simulink model "Irradiance__"  (R2024b)
settings: Solver=ode23  StartTime=0.0  StopTime=1200  RelTol=1e-3
values from neighbouring files (symbols this model uses):
  CellNum = 54    [Inititialisation.m]
  E_g = 1.1    [Inititialisation.m]
  G_ref = 1000    [Inititialisation.m]
  I_sc = 8.21    [Inititialisation.m]
  k_Boltz = 1.380649e-23    [Inititialisation.m]
  K_Isc = 0.0032    [Inititialisation.m]
  K_Vsc = -0.1230    (= -0.123)    [Inititialisation.m]
  LookupR = readmatrix("Data_Out.xlsx", Sheet="Lookup")    [Inititialisation.m]
  n = 0.64611    [Inititialisation.m]
  Num_Paral = 1    [Inititialisation.m]
  NumSeries = 1    [Inititialisation.m]
  q = 1.60217663e-19    [Inititialisation.m]
  R_p = 65.4647    [Inititialisation.m]
  R_s = 0.47804    [Inititialisation.m]
  T_ref = 25+273.15    (= 298.15)    [Inititialisation.m]
  V_oc = 32.9    [Inititialisation.m]
undefined symbols (not defined in the file or in its folder): X, Y, Z
libraries: simulink_extras x10, WormAndGearConstraintLibrary x6, sm_lib x4, nesl_utility x3, fl_lib x2, SignalEditorBlockLib x1
settings Model: Creator=Harrison  LastModifiedBy=Harrison
settings SolverCC: ZeroCrossAlgorithm=Adaptive
settings DebuggingCC: IgnoredZcDiagnostic=none
settings ExplorerConfigSet: InternalSimMechanicsExplorerSettings="<ExplorerConfiguration><canonicalview>default</canonicalview><AnimationSetting><BasePlaybackSpeed>1.0</BasePlaybackSpeed><PlaybackSpeedFactor>0.00390625</PlaybackSpeedFactor></AnimationSetting><TilePanel><TileInfo><Tiles Columns=\"1\" Count=\"1\" Rows=\"1\"><Column Weight=\"1\"/><Row Weight=\"1\"/><Tile Height=\"1\" Width=\"1\" X=\"0\" Y=\"0\"/></Tiles></TileInfo><SceneInfo><SceneViewer><BGColor><R>0.60000002384185791</R><G>0.60000002384185791</G><B>0.60000002384185791</B></BGColor><Camera><DoPerspective>off</DoPerspective><Position><X>0.904674596207072468</X><Y>-1.01398600552732976</Y><Z>1.30819149571960591</Z></Position><Center><X>0.0315254730978809794</X><Y>0.0558159470207882369</Y><Z>0.923626353226344343</Z></Center><Up><X>-0.146611699468769036</X><Y>0.226481916389170257</Y><Z>0.962917935821930748</Z></Up><ViewLimDist>1</ViewLimDist><YLim>0.98754073208570492</YLim><XLim>0.758290204994380601</XLim></Camera></SceneViewer></SceneInfo></TilePanel><MechEditorPanel><Cameras/><GfxPanelCameraMap/><VideoCreator><PlaybackSpeedRatio>0.00115740</PlaybackSpeedRatio><FrameRate>60</FrameRate><VideoFormat>MPEG-4</VideoFormat><FrameSize>auto</FrameSize></VideoCreator></MechEditorPanel></ExplorerConfiguration>"

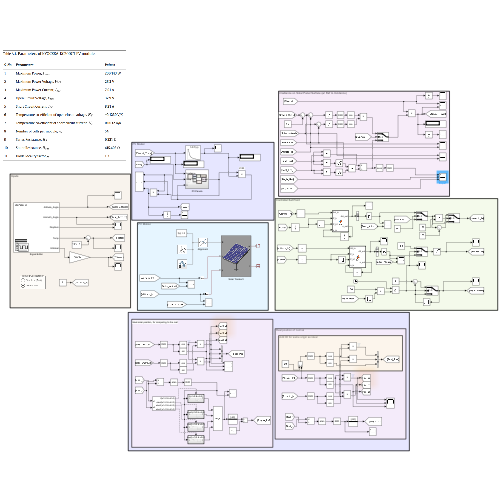
[thumbnail: Simulink's stored preview of the top-level diagram]
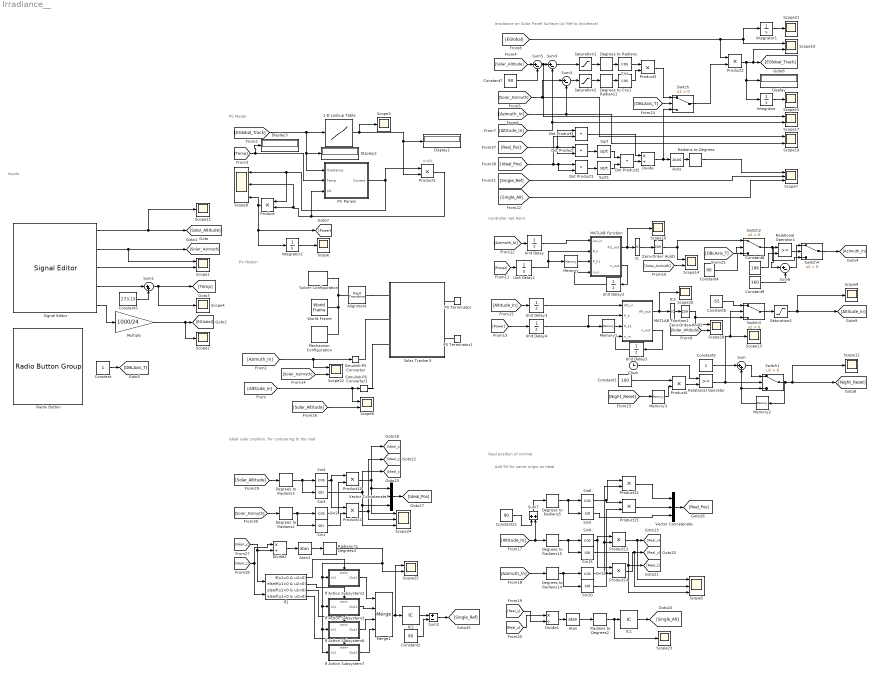
== system Irradiance__ ==
  note: Irradiance on Solar Panel Surface (w/ Ref to Incidence)
  note: Controller Set Point
  note: V=IR
  note: Inputs
  note: PV Motion
  note: PV Model
  note: Ideal solar position, for comparing to the real
  note: Add 90 for same origin as ideal
  note: Real position of normal
  1-D Lookup Table : Lookup_n-D  NumberOfTableDimensions=1  BreakpointsForDimension1=[LookupR(:,1)]  Table=[LookupR(:,2)]  InternalRulePriority=Speed  RndMeth=Simplest
  Acos : Trigonometry  Operator=acos
  Alignment : sm_lib/Frames and Transforms/Rigid Transform  RotationMethod=AlignedAxes  FollAlignAxisA=+Z  BaseAlignAxisA=+Z  FollAlignAxisB=+Y  BaseAlignAxisB=-X  RotationStandardAxis=+Z  RotationAngle=0.0  RotationAngleUnits=deg  RotationArbitraryAxis=[0 0 1]  RotationSequenceAxes=FollowerAxes  RotationSequence=XYX  RotationSequenceAngles=[0 0 0]  RotationSequenceAnglesUnits=deg  RotationMatrix=[1 0 0; 0 1 0; 0 0 1]  Quaternion=[1 0 0 0]  TranslationMethod=None  TranslationCartesianOffset=[0 0 0]  TranslationCartesianOffsetUnits=m  TranslationStandardAxis=+Z  TranslationStandardOffset=0  TranslationStandardOffsetUnits=m  TranslationROffset=0  TranslationROffsetUnits=m  TranslationThetaOffset=0  TranslationThetaOffsetUnits=deg  TranslationZOffset=0  TranslationZOffsetUnits=m
  Atan : Trigonometry  Operator=atan
  Atan1 : Trigonometry  Operator=atan
  Clock : Clock
  Constant : Constant
  Constant1 : Constant  Value=100
  Constant{2,4,7,21} (4 alike) : Constant  Value=90
  Constant3 : Constant  Value=273.15
  Constant5 : Constant
  Constant6 : Constant  Value=-55
  Constant8 : Constant  Value=186
  Constant9 : Constant  Value=360
  Cos : Trigonometry  Operator=cos
  Cos1 : Trigonometry  Operator=cos
  Degrees to Radians{,1..3,5,14..15} (7 alike) : simulink_extras/Transformations/Degrees to Radians
  Display{,1..3} (4 alike) : Display
  Divide : Product  Inputs=*/
  Divide1 : Product  Inputs=*/
  Divide2 : Product  Inputs=*/
  Dot Product{,1..3} (4 alike) : DotProduct  OutDataTypeStr=Inherit: Inherit via internal rule
  IC : InitialCondition  Value=0
  IC1 : InitialCondition  Value=-60
  IC2 : InitialCondition  Value=-60
  IC3 : InitialCondition  Value=-60
  If Action Subsystem2 : Subsystem  TreatAsAtomicUnit=on
  If Action Subsystem3 : Subsystem  TreatAsAtomicUnit=on
  If Action Subsystem6 : Subsystem  TreatAsAtomicUnit=on
  If Action Subsystem7 : Subsystem  TreatAsAtomicUnit=on
  If1 : If  NumInputs=2  IfExpression=u1>0 & u2>0  ElseIfExpressions=u1>0 & u2<0, u1<0 & u2<0, u1<0 & u2>0  ShowElse=off
  Integrator : Integrator
  Integrator1 : Integrator
  Integrator2 : Integrator
  MATLAB Function : MATLAB Function  TreatAsAtomicUnit=on
  MATLAB Function1 : MATLAB Function  TreatAsAtomicUnit=on
  Mechanism Configuration : sm_lib/Utilities/Mechanism Configuration  UniformGravity=Constant  GravityVector=[0 0 -9.80665]  GravityVectorUnits=m/s^2  LinearizationDelta=0.001  JointModeTransitionNonlinearIterations=2
  Memory : Memory
  Memory1 : Memory
  Memory2 : Memory  InitialCondition=1
  Memory3 : Memory  InitialCondition=1
  Merge1 : Merge  Inputs=4
  Multiply : Gain  Gain=1000/24
  PS Terminator : fl_lib/Physical Signals/Sinks/PS Terminator
  PS Terminator1 : fl_lib/Physical Signals/Sinks/PS Terminator
  PV Panels : Subsystem
  Product{,1..4,10..15} (11 alike) : Product
  Radians to Degrees : simulink_extras/Transformations/Radians to Degrees
  Radians to Degrees2 : simulink_extras/Transformations/Radians to Degrees
  Radians to Degrees3 : simulink_extras/Transformations/Radians to Degrees
  Radio Button : RadioButtonGroup  LabelPosition=Hide  SelectedLabel=Double Axis  ButtonGroupName=Tracking Configuration
      settings: Values={{'One Axis (E-W)', 'Double Axis'}, [0 1]}
  Relational Operator : RelationalOperator  OutDataTypeStr=boolean  RndMeth=Simplest  InputSameDT=off
  Relational Operator1 : RelationalOperator  OutDataTypeStr=boolean  RndMeth=Simplest  InputSameDT=off
  Saturation1 : Saturate  UpperLimit=90  LowerLimit=-90
  Saturation2 : Saturate  UpperLimit=90  LowerLimit=-90
  Saturation4 : Saturate  UpperLimit=60  LowerLimit=-60
  Scope{,2..4,9,11..13,15..16,20..21,23} (13 alike) : Scope
  Scope{1,6,10,14,17..19,22,25} (9 alike) : Scope  NumInputPorts=2
  Scope{5,7..8,24} (4 alike) : Scope  NumInputPorts=3
  Signal Editor : SignalEditorBlockLib/Signal Editor  FileName=C:\Users\Harrison\OneDrive\Documents\from 2021\Uni\University\Year 3\Final Year Project\Models\SimOutputs\All_Scenario.mat  ActiveScenario=Scenario_3  ActiveSignal=Altitude_Angle  IsBus=off  OutputBusObjectStr=Bus: BusObject  SampleTime=0  Interpolate=off  ZeroCross=off  OutputAfterFinalValue=Setting to zero  Unit=inherit  PreserveSignalName=on  ApplySigPropsToAllScenarios=on  ApplySigPropsToAllSignals=off
  Simulink-PS Converter : nesl_utility/Simulink-PS Converter  PhysicalDomain=network_engine_domain  SubClassName=ps_input  LeftPortType=input  RightPortType=output  PseudoPeriodic=off  Frequencies=[]  NoiseDistribution=none  NoiseParameters=[]  Unit=deg  AffineConversion=off  FilteringAndDerivatives=filter  SimscapeFilterOrder=2  InputFilterTimeConstant=0.001  UdotUserProvided=0
  Simulink-PS Converter1 : nesl_utility/Simulink-PS Converter  PhysicalDomain=network_engine_domain  SubClassName=ps_input  LeftPortType=input  RightPortType=output  PseudoPeriodic=off  Frequencies=[]  NoiseDistribution=none  NoiseParameters=[]  Unit=deg  AffineConversion=off  FilteringAndDerivatives=filter  SimscapeFilterOrder=2  InputFilterTimeConstant=0.001  UdotUserProvided=0
  Sin{1,3,5,10,15} (5 alike) : Trigonometry
  Sin{2,4,6,9,11} (5 alike) : Trigonometry  Operator=cos
  Solar Tracker3 : Subsystem
      mask Display:
      | image(fullfile('WormAndGearConstraintSupport','Images','SolarTracker.png'));
      | port_label('lconn',1,'B');
      | port_label('lconn',2,'y');
      | port_label('lconn',3,'p');
      | port_label('rconn',1,'w');
      | port_label('rconn',2,'t');
  Solver Configuration : nesl_utility/Solver Configuration  PhysicalDomain=network_engine_domain  SubClassName=solver  LeftPortType=input  RightPortType=generic  Tones=[]  Harmonics=[]  SimulateNoise=off  Profile=off  UseLocalSampling=off  EnableSwitchedLinearOptims=on  FrequencyDomain=off  UseCCode=off  RelTol=0.001  AbsTol=1e-06  MinStep=1e-09  ToWorkspace=off  RevertToSquareIcSolve=off  NumHomotopyIterations=100  PhasorMode=off  PhasorModeNumHarmonics=1  ConsistencySolver=NEWTON_FTOL  IndexReductionMethod=DerivativeReplacement  DoDC=off  ResidualTolerance=1e-09  ConsistencyTolSource=GLOBAL  ConsistencyAbsTol=0.001  ConsistencyRelTol=0.001  ConsistencyTolFactor=0.001  UseLocalSolver=off  LocalSolverChoice=NE_BACKWARD_EULER_ADVANCER  ResolveIndetEquations=on  FunctionEvalNumThread=1  LocalSolverSampleTime=0.001  DoFixedCost=off  MaxNonlinIter=3  MaxModeIter=2  ComputeImpulses=off  ImpulseIterations=2  LinearAlgebra=Sparse  LinearAlgebraNumThread=0  EquationFormulation=NE_TIME_EF  DelaysMemoryBudget=1024  AutomaticFiltering=on  FilteringTimeConstant=0.001  PartitionStorageMethod=AS_NEEDED  PartitionMemoryBudget=1024  PartitionMethod=FAST  MultibodyUseLocalSolver=off  MultibodyLocalSolverChoice=ODE1  MultibodyLocalSolverSampleTime=0.001
  Sqrt : Sqrt
  Sqrt1 : Sqrt
  Sum : Sum  Inputs=|++
  Sum1 : Sum  Inputs=|++
  Sum2 : Sum  Inputs=+-
  Sum{3..6} (4 alike) : Sum  Inputs=|+-
  Sum7 : Sum
  Switch{,1..4} (5 alike) : Switch  Criteria=u2 > Threshold  SaturateOnIntegerOverflow=off  InputSameDT=off
  Unit Delay : UnitDelay  SampleTime=0.015  HasFrameUpgradeWarning=on
  Unit Delay1 : UnitDelay  SampleTime=0.015  HasFrameUpgradeWarning=on
  Unit Delay2 : UnitDelay  SampleTime=0.015  HasFrameUpgradeWarning=on
  Unit Delay3 : UnitDelay  SampleTime=0.01  HasFrameUpgradeWarning=on
  Unit Delay4 : UnitDelay  SampleTime=0.01  HasFrameUpgradeWarning=on
  Unit Delay5 : UnitDelay  SampleTime=0.01  HasFrameUpgradeWarning=on
  Vector Concatenate : Concatenate  NumInputs=3
  Vector Concatenate1 : Concatenate  NumInputs=3
  World Frame : sm_lib/Frames and Transforms/World Frame
  Zero-Order Hold1 : ZeroOrderHold  SampleTime=0.015
  Zero-Order Hold2 : ZeroOrderHold  SampleTime=0.01
  wires:
  Product1/1 -> PV Panels/3(In1), Scope8/2, Product/2
  PV Panels/1(Current) -> Product1/1, Product/1, Scope8/1
  Constant3/1 -> Sum1/2
  [Azimuth_In] -> Scope22/1, Simulink-PS Converter/1
  Multiply/1 -> [EGlobal], Scope2/1
  Sum1/1 -> [Temp], Scope4/1
  [EGlobal_Track] -> 1-D Lookup Table/1, Display2/1, PV Panels/1(Irradiance)
  [Temp] -> Display3/1, PV Panels/2(Temp)
  Signal Editor/2 -> [Solar_Azimuth], Scope1/1
  Signal Editor/3 -> Scope1/2
  Signal Editor/5 -> Multiply/1
  Signal Editor/4 -> Sum1/1
  1-D Lookup Table/1 -> Scope3/1, Product1/2, Display1/1
  Cos/1 -> Product3/1
  Cos1/1 -> Product3/2
  [EGlobal] -> Integrator1/1, Scope10/1, Product2/1
  Degrees to Radians/1 -> Cos/1
  Degrees to Radians1/1 -> Cos1/1
  Memory/1 -> MATLAB Function/3(P_k1)
  MATLAB Function/1(Azi_out) -> Scope16/1, IC/1
  Product/1 -> Integrator2/1, [Power], Scope8/3
  Product2/1 -> Scope10/2, [EGlobal_Track], Integrator/1, Display/1
  [Solar_Azimuth] -> Sum4/1, Scope19/1
  [Azimuth_In] -> Scope19/2, Sum4/2
  [Altitude_In] -> Sum3/2, Scope17/2
  Signal Editor/1 -> Scope11/1, [Solar_Altitude]
  Sum4/1 -> Saturation2/1
  Sum3/1 -> Saturation1/1
  Saturation2/1 -> Degrees to Radians1/1
  Saturation1/1 -> Degrees to Radians/1
  Unit Delay2/1 -> MATLAB Function/4(n_in)
  Unit Delay5/1 -> MATLAB Function1/4(n_in)
  MATLAB Function1/1(Alt_out) -> IC3/1, Scope20/1
  Memory1/1 -> MATLAB Function1/3(P_k1)
  [Altitude_In] -> Scope6/1, Simulink-PS Converter1/1
  [Azimuth_In] -> Unit Delay/1
  Unit Delay/1 -> MATLAB Function/1(Azi_in)
  Unit Delay1/1 -> MATLAB Function/2(P_k), Memory/1
  MATLAB Function/2(n_out) -> Unit Delay2/1
  [Power] -> Unit Delay1/1
  IC/1 -> Zero-Order Hold1/1
  Zero-Order Hold1/1 -> Scope14/1, Switch2/1
  [Solar_Azimuth] -> Scope14/2
  [Power] -> Unit Delay4/1
  Unit Delay4/1 -> MATLAB Function1/2(P_k), Memory1/1
  MATLAB Function1/2(n_out) -> Unit Delay5/1
  IC3/1 -> Zero-Order Hold2/1
  [Solar_Altitude] -> Scope18/2
  [Solar_Azimuth] -> Scope22/2
  [Solar_Altitude] -> Scope6/2
  [Real_y] -> Divide1/2
  [Ideal_y] -> Divide2/2, If1/1
  [Azimuth_In] -> Degrees to Radians14/1
  If Action Subsystem3/1(Out1) -> Merge1/2
  Degrees to Radians2/1 -> Sin2/1, Sin1/1
  Atan1/1 -> Radians to Degrees3/1
  Constant21/1 -> Sum7/1
  If Action Subsystem2/1(Out1) -> Merge1/1
  Merge1/1 -> IC2/1, Scope25/1
  Divide2/1 -> Atan1/1
  Radians to Degrees2/1 -> IC1/1, Scope23/1
  Product15/1 -> Vector Concatenate/2
  Divide1/1 -> Atan/1
  Vector Concatenate1/1 -> [Ideal_Pos]
  If Action Subsystem7/1(Out1) -> Merge1/4
  IC2/1 -> Sum2/1
  [Solar_Altitude] -> Degrees to Radians3/1
  Product13/1 -> Scope5/1, [Real_x]
  [Real_z] -> Divide1/1
  Sum7/1 -> Degrees to Radians5/1
  If1/3 -> If Action Subsystem6/Action
  Sin9/1 -> Product13/1, Product14/1
  [Solar_Azimuth] -> Degrees to Radians2/1
  Degrees to Radians15/1 -> Sin15/1, Sin9/1
  Sin3/1 -> Scope24/3, Vector Concatenate1/3, [Ideal_z]
  If Action Subsystem6/1(Out1) -> Merge1/3
  Radians to Degrees3/1 -> If Action Subsystem2/1(In1), If Action Subsystem3/1(In1), If Action Subsystem6/1(In1), If Action Subsystem7/1(In1), Scope25/2
  Sin11/1 -> Product13/2, Product12/2
  [Ideal_z] -> Divide2/1, If1/2
  Product12/1 -> Vector Concatenate/1
  If1/2 -> If Action Subsystem3/Action
  Product11/1 -> [Ideal_y], Vector Concatenate1/2, Scope24/2
  Atan/1 -> Radians to Degrees2/1
  Degrees to Radians5/1 -> Sin6/1, Sin5/1
  Sin1/1 -> Product11/2
  Product14/1 -> Scope5/2, [Real_y]
  Sum2/1 -> [Single_Ref]
  Sin15/1 -> Scope5/3, [Real_z]
  If1/4 -> If Action Subsystem7/Action
  Sin4/1 -> Product11/1, Product10/1
  Sin10/1 -> Product15/2, Product14/2
  Degrees to Radians3/1 -> Sin4/1, Sin3/1
  IC1/1 -> [Single_Alt]
  If1/1 -> If Action Subsystem2/Action
  Constant2/1 -> Sum2/2
  Sin5/1 -> Vector Concatenate/3
  Degrees to Radians14/1 -> Sin10/1, Sin11/1
  Sin2/1 -> Product10/2
  [Altitude_In] -> Sum7/2, Degrees to Radians15/1
  Product10/1 -> Vector Concatenate1/1, Scope24/1, [Ideal_x]
  Sin6/1 -> Product15/1, Product12/1
  Vector Concatenate/1 -> [Real_Pos]
  Sqrt1/1 -> Dot Product2/2
  Dot Product3/1 -> Divide/1
  Dot Product/1 -> Sqrt/1
  [Ideal_Pos] -> Dot Product3/2, Dot Product1/1, Dot Product1/2
  Dot Product1/1 -> Sqrt1/1
  Dot Product2/1 -> Divide/2
  Sqrt/1 -> Dot Product2/1
  [Real_Pos] -> Dot Product3/1, Dot Product/2, Dot Product/1
  Product3/1 -> Switch/1
  Switch/1 -> Product2/2
  Divide/1 -> Switch/3, Acos/1
  [DBLAxis_T] -> Switch/2
  Acos/1 -> Radians to Degrees/1
  Radians to Degrees/1 -> Scope7/1
  [Single_Ref] -> Scope7/2
  [Single_Alt] -> Scope7/3
  Constant/1 -> [DBLAxis_T]
  [Altitude_In] -> Unit Delay3/1
  Unit Delay3/1 -> MATLAB Function1/1(Alt_in)
  Zero-Order Hold2/1 -> Scope18/1, Switch3/3
  Constant4/1 -> Switch2/3
  [DBLAxis_T] -> Switch2/2
  Switch2/1 -> Switch4/3, Sum6/1, Relational Operator1/1
  Constant1/1 -> Product4/1
  Product4/1 -> Relational Operator/2
  Clock/1 -> Relational Operator/1
  Constant5/1 -> Sum/1
  Switch1/1 -> Memory2/1, Scope12/1, [Night_Reset]
  Memory2/1 -> Switch1/3, Sum/2
  Sum/1 -> Switch1/1
  [Night_Reset] -> Memory3/1
  Relational Operator/1 -> Switch1/2, Scope13/1, Switch3/2
  Memory3/1 -> Product4/2
  Switch3/1 -> Saturation4/1
  Constant6/1 -> Switch3/1
  Saturation4/1 -> Scope9/1, [Altitude_In]
  Sum5/1 -> Scope17/1, Sum3/1
  [Solar_Altitude] -> Sum5/1
  Constant7/1 -> Sum5/2
  Integrator/1 -> Scope15/1
  Integrator1/1 -> Scope21/1
  Integrator2/1 -> Scope/1
  Constant8/1 -> Relational Operator1/2
  Relational Operator1/1 -> Switch4/2
  Switch4/1 -> [Azimuth_In]
  Constant9/1 -> Sum6/2
  Sum6/1 -> Switch4/1
  connections:
  Mechanism Configuration/RConn1 -- World Frame/RConn1 -- Solver Configuration/RConn1 -- Alignment/LConn1
  Simulink-PS Converter1/RConn1 -- Solar Tracker3/LConn3
  Simulink-PS Converter/RConn1 -- Solar Tracker3/LConn2
  Alignment/RConn1 -- Solar Tracker3/LConn1
  PS Terminator/LConn1 -- Solar Tracker3/RConn1
  PS Terminator1/LConn1 -- Solar Tracker3/RConn2

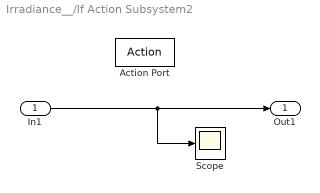
== system Irradiance__/If Action Subsystem2 ==
  In1 : Inport
  Action Port : ActionPort  ActionPortLabel=if(u1>0 & u2>0)
  Scope : Scope
  Out1 : Outport
  wires:
  In1/1 -> Out1/1, Scope/1

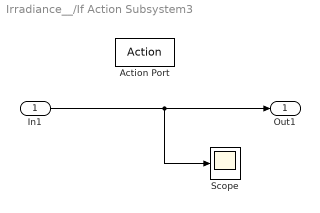
== system Irradiance__/If Action Subsystem3 ==
  In1 : Inport
  Action Port : ActionPort  ActionPortLabel=elseif(u1>0 & u2<0)
  Scope : Scope
  Out1 : Outport
  wires:
  In1/1 -> Out1/1, Scope/1

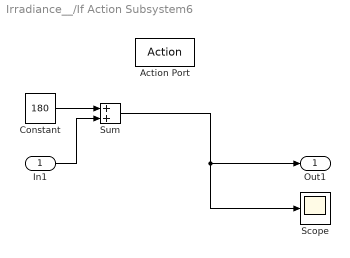
== system Irradiance__/If Action Subsystem6 ==
  In1 : Inport
  Action Port : ActionPort  ActionPortLabel=elseif( u1<0 & u2<0)
  Constant : Constant  Value=180
  Scope : Scope
  Sum : Sum
  Out1 : Outport
  wires:
  Sum/1 -> Out1/1, Scope/1
  Constant/1 -> Sum/1
  In1/1 -> Sum/2

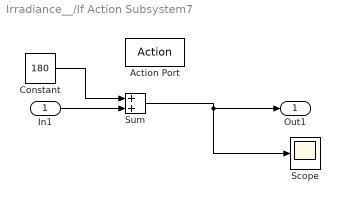
== system Irradiance__/If Action Subsystem7 ==
  In1 : Inport
  Action Port : ActionPort  ActionPortLabel=elseif( u1<0 & u2>0)
  Constant : Constant  Value=180
  Scope : Scope
  Sum : Sum
  Out1 : Outport
  wires:
  Sum/1 -> Out1/1, Scope/1
  In1/1 -> Sum/2
  Constant/1 -> Sum/1

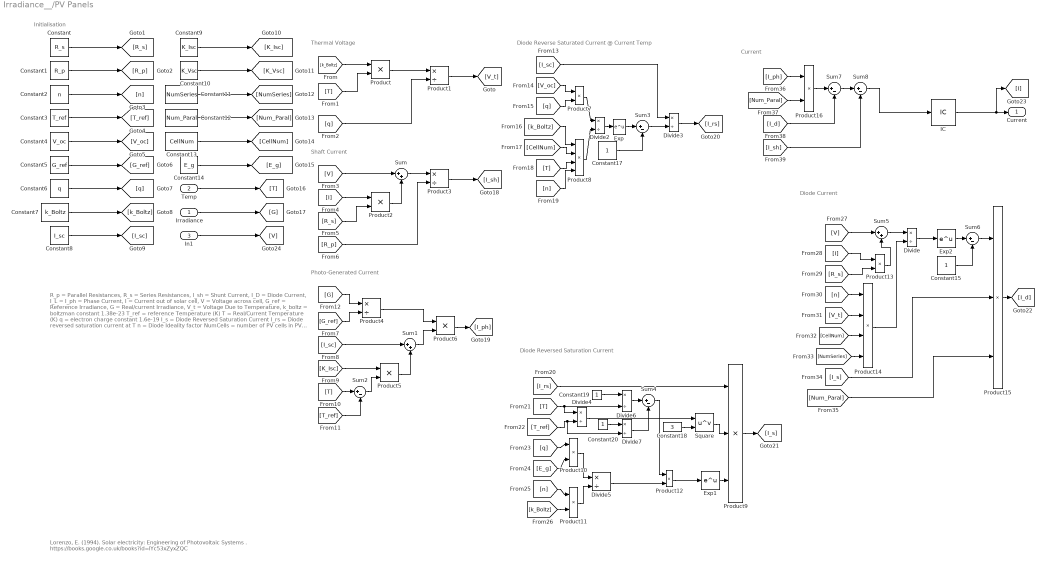
== system Irradiance__/PV Panels ==
  note: R_p = Parallel Resistances,
      | R_s = Series Resistances,
      | I_sh = Shunt Current,
      | I_D = Diode Current,
      | I_L = I_ph = Phase Current,
      | I = Current out of solar cell,
      | V = Voltage across cell,
      | G_ref = Reference Irradiance,
      | G = Real/current Irradiance,
      | V_t = Voltage Due to Temperature,
      | k_boltz = boltzman constant 1.38e-23
      | T_ref = reference Temperature (K)
      | T = Real/Current Temperature (K)
      | q = electron charge constant 1.6e-19
      | I_s = Diode Reversed Saturation Current
      | I_rs = Diode reversed saturation current at T
      | n = Diode Ideality factor
      | NumCells = number of PV cells in PV panel,
      | NumSeries = Number of PV panels in series,
      | Num_Paral = Number of PV panels in parallel,
      | E_g = Band gap energy of the cell, 1.12eV
  note: Lorenzo, E. (1994). Solar electricity: Engineering of Photovoltaic Systems . https://books.google.co.uk/books?id=lYc53xZyxZQC
  note: Initialisation
  note: Current
  note: Diode Current
  note: Diode Reversed Saturation Current
  note: Diode Reverse Saturated Current @ Current Temp
  note: Photo-Generated Current
  note: Shaft Current
  note: Thermal Voltage
  Irradiance : Inport
  Temp : Inport  Port=2
  In1 : Inport  Port=3
  Constant : Constant  Value=R_s
  Constant1 : Constant  Value=R_p
  Constant10 : Constant  Value=K_Vsc
  Constant11 : Constant  Value=NumSeries
  Constant12 : Constant  Value=Num_Paral
  Constant13 : Constant  Value=CellNum
  Constant14 : Constant  Value=E_g
  Constant{15,17,19..20} (4 alike) : Constant
  Constant18 : Constant  Value=3
  Constant2 : Constant  Value=n
  Constant3 : Constant  Value=T_ref
  Constant4 : Constant  Value=V_oc
  Constant5 : Constant  Value=G_ref
  Constant6 : Constant  Value=q
  Constant7 : Constant  Value=k_Boltz
  Constant8 : Constant  Value=I_sc
  Constant9 : Constant  Value=K_Isc
  Divide{,2..7} (7 alike) : Product  Inputs=*/
  Exp : Math
  Exp1 : Math
  Exp2 : Math
  IC : InitialCondition  Value=0
  Product{,2,5..7,10..13,16} (10 alike) : Product
  Product1 : Product  Inputs=*/
  Product14 : Product  Inputs=4
  Product15 : Product  Inputs=3
  Product3 : Product  Inputs=*/
  Product4 : Product  Inputs=*/
  Product8 : Product  Inputs=4
  Product9 : Product  Inputs=3
  Square : Math  Operator=pow
  Sum : Sum  Inputs=|++
  Sum1 : Sum  Inputs=|++
  Sum{2..4,6..8} (6 alike) : Sum  Inputs=|+-
  Sum5 : Sum  Inputs=|++
  Current : Outport
  wires:
  [k_Boltz] -> Product/1
  [T] -> Product/2
  Product/1 -> Product1/1
  [q] -> Product1/2
  Product1/1 -> [V_t]
  Constant/1 -> [R_s]
  Constant1/1 -> [R_p]
  Constant2/1 -> [n]
  Constant3/1 -> [T_ref]
  Constant4/1 -> [V_oc]
  Constant5/1 -> [G_ref]
  Constant6/1 -> [q]
  Constant7/1 -> [k_Boltz]
  Constant8/1 -> [I_sc]
  Constant9/1 -> [K_Isc]
  Constant12/1 -> [Num_Paral]
  Constant10/1 -> [K_Vsc]
  Constant13/1 -> [CellNum]
  Constant11/1 -> [NumSeries]
  Constant14/1 -> [E_g]
  Temp/1 -> [T]
  Irradiance/1 -> [G]
  [R_s] -> Product2/2
  Product2/1 -> Sum/2
  Sum/1 -> Product3/1
  [R_p] -> Product3/2
  Product3/1 -> [I_sh]
  [G] -> Product4/1
  [G_ref] -> Product4/2
  [I_sc] -> Sum1/1
  [K_Isc] -> Product5/1
  [T] -> Sum2/1
  [T_ref] -> Sum2/2
  Sum2/1 -> Product5/2
  Product5/1 -> Sum1/2
  Sum1/1 -> Product6/2
  Product4/1 -> Product6/1
  Product6/1 -> [I_ph]
  [V_oc] -> Product7/1
  [q] -> Product7/2
  [k_Boltz] -> Product8/1
  [CellNum] -> Product8/2
  [T] -> Product8/3
  [n] -> Product8/4
  Product7/1 -> Divide2/1
  Product8/1 -> Divide2/2
  Divide2/1 -> Exp/1
  Exp/1 -> Sum3/1
  Constant17/1 -> Sum3/2
  Sum3/1 -> Divide3/2
  [I_sc] -> Divide3/1
  Divide3/1 -> [I_rs]
  [T] -> Divide4/1, Divide6/2
  [T_ref] -> Divide7/2, Divide4/2
  Constant18/1 -> Square/2
  Divide4/1 -> Square/1
  [I_rs] -> Product9/1
  Square/1 -> Product9/2
  Exp1/1 -> Product9/3
  [q] -> Product10/1
  [E_g] -> Product10/2
  [n] -> Product11/1
  [k_Boltz] -> Product11/2
  Product10/1 -> Divide5/1
  Product11/1 -> Divide5/2
  Constant19/1 -> Divide6/1
  Constant20/1 -> Divide7/1
  Divide6/1 -> Sum4/1
  Divide7/1 -> Sum4/2
  Divide5/1 -> Product12/2
  Sum4/1 -> Product12/1
  Product12/1 -> Exp1/1
  Product9/1 -> [I_s]
  [R_s] -> Product13/2
  Product13/1 -> Sum5/2
  Sum5/1 -> Divide/1
  [n] -> Product14/1
  [V_t] -> Product14/2
  [CellNum] -> Product14/3
  [NumSeries] -> Product14/4
  Product14/1 -> Divide/2
  Divide/1 -> Exp2/1
  Exp2/1 -> Sum6/1
  Constant15/1 -> Sum6/2
  Sum6/1 -> Product15/1
  [Num_Paral] -> Product15/3
  [I_s] -> Product15/2
  Product15/1 -> [I_d]
  [I_ph] -> Product16/1
  [Num_Paral] -> Product16/2
  Product16/1 -> Sum7/1
  [I_d] -> Sum7/2
  Sum7/1 -> Sum8/1
  [I_sh] -> Sum8/2
  [V] -> Sum/1
  [V] -> Sum5/1
  In1/1 -> [V]
  [I] -> Product2/1
  [I] -> Product13/1
  Sum8/1 -> IC/1
  IC/1 -> [I], Current/1

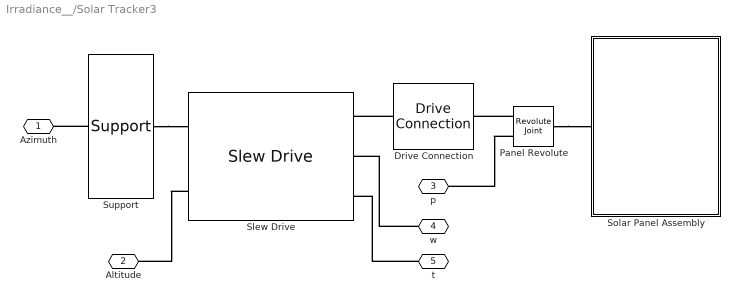
== system Irradiance__/Solar Tracker3 ==
  Drive Connection : WormAndGearConstraintLibrary/Drive Connection  connRadius=driveconn.connectionRadius  connThickness=driveconn.connectionThickness  connLength=driveconn.connectionLength  bracketWidth=driveconn.bracketWidthHeight  bracketThickness=driveconn.bracketThickness  holeRadius=driveconn.holeRadius  holeOffset=driveconn.holeOffset  baseThickness=driveconn.baseThickness  rho=driveconn.density  color=driveconn.color
  Panel Revolute : sm_lib/Joints/Revolute Joint  JointMode=Normal  CompositeWrenchDir=FollowerOnBase  CompositeWrenchFrame=BaseFrame  SenseConstraintForce=off  SenseConstraintTorque=off  SenseTotalForce=off  SenseTotalTorque=off  PositionTargetSpecify=on  PositionTargetPriority=High  PositionTargetValue=panelrevolute.q0  PositionTargetValueUnits=deg  VelocityTargetSpecify=off  VelocityTargetPriority=High  VelocityTargetValue=0  VelocityTargetValueUnits=deg/s  EquilibriumPosition=0  EquilibriumPositionUnits=deg  SpringStiffness=0  SpringStiffnessUnits=N*m/deg  DampingCoefficient=0  DampingCoefficientUnits=N*m/(deg/s)  LowerLimitSpecify=off  LowerLimitBound=-90  LowerLimitBoundUnits=deg  LowerLimitStiffness=1e4  LowerLimitStiffnessUnits=N*m/deg  LowerLimitDamping=10  LowerLimitDampingUnits=N*m/(deg/s)  LowerLimitTransitionRegionWidth=0.1  LowerLimitTransitionRegionWidthUnits=deg  UpperLimitSpecify=off  UpperLimitBound=90  UpperLimitBoundUnits=deg  UpperLimitStiffness=1e4  UpperLimitStiffnessUnits=N*m/deg  UpperLimitDamping=10  UpperLimitDampingUnits=N*m/(deg/s)  UpperLimitTransitionRegionWidth=0.1  UpperLimitTransitionRegionWidthUnits=deg  TorqueActuationMode=ComputedTorque  MotionActuationMode=InputMotion  SensePosition=off  SenseVelocity=off  SenseAcceleration=off  SenseTorqueForce=off  SenseLowerLimitTorqueForce=off  SenseUpperLimitTorqueForce=off
  Slew Drive : WormAndGearConstraintLibrary/Slew Drive  wormLeadAngle=slewdrive.wormLeadAngle  wormLength=slewdrive.wormLength  gearOuterRadius=slewdrive.gearOuterRadius  gearInnerRadius=slewdrive.gearInnerRadius  gearExposedRadius=slewdrive.gearExposedRadius  ratio=slewdrive.ratio  housingThickness=slewdrive.housingThickness  bWormRevolute=slewdrive.wormRevoluteDamping  wormRho=slewdrive.wormDensity  gearRho=slewdrive.gearDensity  housingRho=slewdrive.housingDensity  wormColor=slewdrive.wormColor  gearColor=slewdrive.gearColor  housingColor=slewdrive.housingColor  housingOpacity=slewdrive.housingOpacity
  Solar Panel Assembly : Subsystem
      mask Display:
      | image(fullfile('WormAndGearConstraintSupport','Images','SolarPanel.png'));
      | port_label('lconn',1,'H');
  Support : WormAndGearConstraintLibrary/Support  columnRadius=support.columnRadius  columnThickness=support.columnThickness  columnHeight=support.columnHeight  baseWidth=support.baseWidth  baseThickness=support.baseThickness  rho=support.density  color=support.color
  Azimuth : PMIOPort  Side=Left
  Altitude : PMIOPort  Port=2  Side=Left
  p : PMIOPort  Port=3  Side=Left
  w : PMIOPort  Port=4  Side=Right
  t : PMIOPort  Port=5  Side=Right
  connections:
  Support/LConn1 -- Azimuth/RConn1
  Support/RConn1 -- Slew Drive/LConn1
  Drive Connection/LConn1 -- Slew Drive/RConn1
  Panel Revolute/LConn1 -- Drive Connection/RConn1
  w/RConn1 -- Slew Drive/RConn2
  Slew Drive/LConn2 -- Altitude/RConn1
  Panel Revolute/LConn2 -- p/RConn1
  Panel Revolute/RConn1 -- Solar Panel Assembly/LConn1
  t/RConn1 -- Slew Drive/RConn3

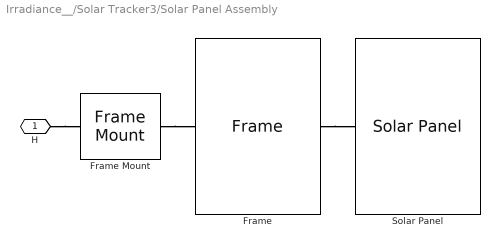
== system Irradiance__/Solar Tracker3/Solar Panel Assembly ==
  Frame : WormAndGearConstraintLibrary/Frame  width=frame.width  height=frame.height  depth=frame.depth  beamWidth=frame.beamWidth  beamThickness=frame.beamThickness  frameWidth=frame.frameWidth  frameThickness=frame.frameThickness  rho=frame.density  beamColor=frame.beamColor  frameColor=frame.frameColor
  Frame Mount : WormAndGearConstraintLibrary/Frame Mount  bracketWidth=framemount.bracketWidthHeight  bracketThickness=framemount.bracketThickness  bracketOffset=framemount.bracketOffset  holeRadius=framemount.holeRadius  holeOffset=framemount.holeOffset  baseThickness=framemount.baseThickness  rho=framemount.density  mountColor=framemount.mountColor  pinColor=framemount.pinColor
  Solar Panel : WormAndGearConstraintLibrary/Solar Panel  width=solarpanel.width  height=solarpanel.height  frameWidth=solarpanel.frameWidth  frameDepth=solarpanel.frameDepth  cellsRho=solarpanel.cellDensity  frameRho=solarpanel.frameDensity  cellsColor=solarpanel.cellColor  frameColor=solarpanel.frameColor
  H : PMIOPort  Side=Left
  connections:
  Frame/RConn1 -- Solar Panel/LConn1
  Frame Mount/LConn1 -- Frame/LConn1
  H/RConn1 -- Frame Mount/RConn1

== matlab function Irradiance__/MATLAB Function1 ==
  data: Alt_in input; Alt_out output; P_k input; P_k1 input; n_in input; n_out output
function [Alt_out, n_out] = fcn(Alt_in, P_k, P_k1, n_in)
if n_in == 0
    n_out = 1;
    Alt_out = Alt_in + 3;
elseif n_in == 1
    if P_k1 < P_k
        Alt_out = Alt_in;
        n_out = 0;
    else
        Alt_out = Alt_in - 6;
        n_out = 2;
    end
elseif n_in == 2
    if P_k > P_k1
        Alt_out = Alt_in;
        n_out = 0;
        ans = "1,2"
    else
        Alt_out = Alt_in + 3;
        n_out = 0;
        ans = "2,2"
    end
else
    Alt_out = Alt_in;
    n_out = n_in;
    ans = "3"
end

== matlab function Irradiance__/MATLAB Function ==
  data: Azi_in input; Azi_out output; P_k input; P_k1 input; n_in input; n_out output
function [Azi_out, n_out] = fcn(Azi_in, P_k, P_k1, n_in)
if n_in == 0
    n_out = 1;
    Azi_out = Azi_in + 3;
elseif n_in == 1
    if P_k1 < P_k
        Azi_out = Azi_in;
        n_out = 0;
    else
        Azi_out = Azi_in - 6;
        n_out = 2;
    end
elseif n_in == 2
    if P_k > P_k1
        Azi_out = Azi_in;
        n_out = 0;
        ans = "1,2"
    else
        Azi_out = Azi_in + 3;
        n_out = 0;
        ans = "2,2"
    end
else
    Azi_out = Azi_in;
    n_out = n_in;
    ans = "3"
end
